simulink model "sm_car_testrig_susp_dwa_hp"  (R2025b)
settings: Solver=ode23t  StartTime=0.0  StopTime=1e-9  RelTol=1e-3  EnableMultiTasking=on
PostLoadFcn:
  | sm_car_load_vehicle_data(bdroot,'016');
undefined symbols (not defined in the file): Init, LAf, LAr, UAf, UAr, Vehicle, X, Y, Z
libraries: sm_lib x102, nesl_utility x67, Suspension_Utilities x8, Linkage_Arms x6, Linkage_DW_A x4, fl_lib x4, Linkage_Shock x2, Linkage_Uprights x2
(part 4 of 4)

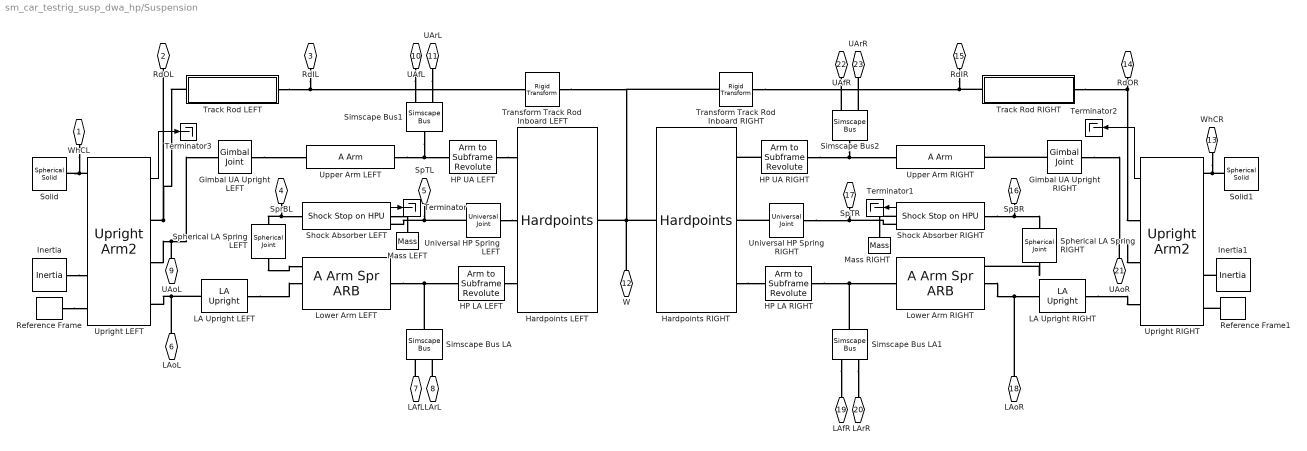
== system sm_car_testrig_susp_dwa_hp/Suspension ==
  Gimbal UA Upright LEFT : sm_lib/Joints/Gimbal Joint  JointMode=Normal  CompositeWrenchDir=FollowerOnBase  CompositeWrenchFrame=BaseFrame  SenseConstraintForce=off  SenseConstraintTorque=off  SenseTotalForce=off  SenseTotalTorque=off  RxPositionTargetSpecify=off  RxPositionTargetPriority=High  RxPositionTargetValue=0  RxPositionTargetValueUnits=deg  RxVelocityTargetSpecify=off  RxVelocityTargetPriority=High  RxVelocityTargetValue=0  RxVelocityTargetValueUnits=deg/s  RxEquilibriumPosition=0  RxEquilibriumPositionUnits=deg  RxSpringStiffness=0  RxSpringStiffnessUnits=N*m/deg  RxDampingCoefficient=0  RxDampingCoefficientUnits=N*m/(deg/s)  RxLowerLimitSpecify=off  RxLowerLimitBound=-90  RxLowerLimitBoundUnits=deg  RxLowerLimitStiffness=1e4  RxLowerLimitStiffnessUnits=N*m/deg  RxLowerLimitDamping=10  RxLowerLimitDampingUnits=N*m/(deg/s)  RxLowerLimitTransitionRegionWidth=0.1  RxLowerLimitTransitionRegionWidthUnits=deg  RxUpperLimitSpecify=off  RxUpperLimitBound=90  RxUpperLimitBoundUnits=deg  RxUpperLimitStiffness=1e4  RxUpperLimitStiffnessUnits=N*m/deg  RxUpperLimitDamping=10  RxUpperLimitDampingUnits=N*m/(deg/s)  RxUpperLimitTransitionRegionWidth=0.1  RxUpperLimitTransitionRegionWidthUnits=deg  RxTorqueActuationMode=NoTorque  RxMotionActuationMode=ComputedMotion  RxSensePosition=off  RxSenseVelocity=off  RxSenseAcceleration=off  RxSenseTorqueForce=off  RxSenseLowerLimitTorqueForce=off  RxSenseUpperLimitTorqueForce=off  RyPositionTargetSpecify=off  RyPositionTargetPriority=Low  RyPositionTargetValue=0  RyPositionTargetValueUnits=deg  RyVelocityTargetSpecify=off  RyVelocityTargetPriority=High  RyVelocityTargetValue=0  RyVelocityTargetValueUnits=deg/s  RyEquilibriumPosition=0  RyEquilibriumPositionUnits=deg  RySpringStiffness=0  RySpringStiffnessUnits=N*m/deg  RyDampingCoefficient=0  RyDampingCoefficientUnits=N*m/(deg/s)  RyLowerLimitSpecify=off  RyLowerLimitBound=-90  RyLowerLimitBoundUnits=deg  RyLowerLimitStiffness=1e4  RyLowerLimitStiffnessUnits=N*m/deg  RyLowerLimitDamping=10  RyLowerLimitDampingUnits=N*m/(deg/s)  RyLowerLimitTransitionRegionWidth=0.1  RyLowerLimitTransitionRegionWidthUnits=deg  RyUpperLimitSpecify=off  RyUpperLimitBound=90  RyUpperLimitBoundUnits=deg  RyUpperLimitStiffness=1e4  RyUpperLimitStiffnessUnits=N*m/deg  RyUpperLimitDamping=10  RyUpperLimitDampingUnits=N*m/(deg/s)  RyUpperLimitTransitionRegionWidth=0.1  RyUpperLimitTransitionRegionWidthUnits=deg  RyTorqueActuationMode=NoTorque  RyMotionActuationMode=ComputedMotion  RySensePosition=off  RySenseVelocity=off  RySenseAcceleration=off  RySenseTorqueForce=off  RySenseLowerLimitTorqueForce=off  RySenseUpperLimitTorqueForce=off  RzPositionTargetSpecify=off  RzPositionTargetPriority=Low  RzPositionTargetValue=90  RzPositionTargetValueUnits=deg  RzVelocityTargetSpecify=off  RzVelocityTargetPriority=High  RzVelocityTargetValue=0  RzVelocityTargetValueUnits=deg/s  RzEquilibriumPosition=0  RzEquilibriumPositionUnits=deg  RzSpringStiffness=0  RzSpringStiffnessUnits=N*m/deg  RzDampingCoefficient=0  RzDampingCoefficientUnits=N*m/(deg/s)  RzLowerLimitSpecify=off  RzLowerLimitBound=-90  RzLowerLimitBoundUnits=deg  RzLowerLimitStiffness=1e4  RzLowerLimitStiffnessUnits=N*m/deg  RzLowerLimitDamping=10  RzLowerLimitDampingUnits=N*m/(deg/s)  RzLowerLimitTransitionRegionWidth=0.1  RzLowerLimitTransitionRegionWidthUnits=deg  RzUpperLimitSpecify=off  RzUpperLimitBound=90  RzUpperLimitBoundUnits=deg  RzUpperLimitStiffness=1e4  RzUpperLimitStiffnessUnits=N*m/deg  RzUpperLimitDamping=10  RzUpperLimitDampingUnits=N*m/(deg/s)  RzUpperLimitTransitionRegionWidth=0.1  RzUpperLimitTransitionRegionWidthUnits=deg  RzTorqueActuationMode=NoTorque  RzMotionActuationMode=ComputedMotion  RzSensePosition=off  RzSenseVelocity=off  RzSenseAcceleration=off  RzSenseTorqueForce=off  RzSenseLowerLimitTorqueForce=off  RzSenseUpperLimitTorqueForce=off
  Gimbal UA Upright RIGHT : sm_lib/Joints/Gimbal Joint  JointMode=Normal  CompositeWrenchDir=FollowerOnBase  CompositeWrenchFrame=BaseFrame  SenseConstraintForce=off  SenseConstraintTorque=off  SenseTotalForce=off  SenseTotalTorque=off  RxPositionTargetSpecify=off  RxPositionTargetPriority=High  RxPositionTargetValue=0  RxPositionTargetValueUnits=deg  RxVelocityTargetSpecify=off  RxVelocityTargetPriority=High  RxVelocityTargetValue=0  RxVelocityTargetValueUnits=deg/s  RxEquilibriumPosition=0  RxEquilibriumPositionUnits=deg  RxSpringStiffness=0  RxSpringStiffnessUnits=N*m/deg  RxDampingCoefficient=0  RxDampingCoefficientUnits=N*m/(deg/s)  RxLowerLimitSpecify=off  RxLowerLimitBound=-90  RxLowerLimitBoundUnits=deg  RxLowerLimitStiffness=1e4  RxLowerLimitStiffnessUnits=N*m/deg  RxLowerLimitDamping=10  RxLowerLimitDampingUnits=N*m/(deg/s)  RxLowerLimitTransitionRegionWidth=0.1  RxLowerLimitTransitionRegionWidthUnits=deg  RxUpperLimitSpecify=off  RxUpperLimitBound=90  RxUpperLimitBoundUnits=deg  RxUpperLimitStiffness=1e4  RxUpperLimitStiffnessUnits=N*m/deg  RxUpperLimitDamping=10  RxUpperLimitDampingUnits=N*m/(deg/s)  RxUpperLimitTransitionRegionWidth=0.1  RxUpperLimitTransitionRegionWidthUnits=deg  RxTorqueActuationMode=NoTorque  RxMotionActuationMode=ComputedMotion  RxSensePosition=off  RxSenseVelocity=off  RxSenseAcceleration=off  RxSenseTorqueForce=off  RxSenseLowerLimitTorqueForce=off  RxSenseUpperLimitTorqueForce=off  RyPositionTargetSpecify=off  RyPositionTargetPriority=Low  RyPositionTargetValue=0  RyPositionTargetValueUnits=deg  RyVelocityTargetSpecify=off  RyVelocityTargetPriority=High  RyVelocityTargetValue=0  RyVelocityTargetValueUnits=deg/s  RyEquilibriumPosition=0  RyEquilibriumPositionUnits=deg  RySpringStiffness=0  RySpringStiffnessUnits=N*m/deg  RyDampingCoefficient=0  RyDampingCoefficientUnits=N*m/(deg/s)  RyLowerLimitSpecify=off  RyLowerLimitBound=-90  RyLowerLimitBoundUnits=deg  RyLowerLimitStiffness=1e4  RyLowerLimitStiffnessUnits=N*m/deg  RyLowerLimitDamping=10  RyLowerLimitDampingUnits=N*m/(deg/s)  RyLowerLimitTransitionRegionWidth=0.1  RyLowerLimitTransitionRegionWidthUnits=deg  RyUpperLimitSpecify=off  RyUpperLimitBound=90  RyUpperLimitBoundUnits=deg  RyUpperLimitStiffness=1e4  RyUpperLimitStiffnessUnits=N*m/deg  RyUpperLimitDamping=10  RyUpperLimitDampingUnits=N*m/(deg/s)  RyUpperLimitTransitionRegionWidth=0.1  RyUpperLimitTransitionRegionWidthUnits=deg  RyTorqueActuationMode=NoTorque  RyMotionActuationMode=ComputedMotion  RySensePosition=off  RySenseVelocity=off  RySenseAcceleration=off  RySenseTorqueForce=off  RySenseLowerLimitTorqueForce=off  RySenseUpperLimitTorqueForce=off  RzPositionTargetSpecify=off  RzPositionTargetPriority=Low  RzPositionTargetValue=90  RzPositionTargetValueUnits=deg  RzVelocityTargetSpecify=off  RzVelocityTargetPriority=High  RzVelocityTargetValue=0  RzVelocityTargetValueUnits=deg/s  RzEquilibriumPosition=0  RzEquilibriumPositionUnits=deg  RzSpringStiffness=0  RzSpringStiffnessUnits=N*m/deg  RzDampingCoefficient=0  RzDampingCoefficientUnits=N*m/(deg/s)  RzLowerLimitSpecify=off  RzLowerLimitBound=-90  RzLowerLimitBoundUnits=deg  RzLowerLimitStiffness=1e4  RzLowerLimitStiffnessUnits=N*m/deg  RzLowerLimitDamping=10  RzLowerLimitDampingUnits=N*m/(deg/s)  RzLowerLimitTransitionRegionWidth=0.1  RzLowerLimitTransitionRegionWidthUnits=deg  RzUpperLimitSpecify=off  RzUpperLimitBound=90  RzUpperLimitBoundUnits=deg  RzUpperLimitStiffness=1e4  RzUpperLimitStiffnessUnits=N*m/deg  RzUpperLimitDamping=10  RzUpperLimitDampingUnits=N*m/(deg/s)  RzUpperLimitTransitionRegionWidth=0.1  RzUpperLimitTransitionRegionWidthUnits=deg  RzTorqueActuationMode=NoTorque  RzMotionActuationMode=ComputedMotion  RzSensePosition=off  RzSenseVelocity=off  RzSenseAcceleration=off  RzSenseTorqueForce=off  RzSenseLowerLimitTorqueForce=off  RzSenseUpperLimitTorqueForce=off
  HP LA LEFT : Suspension_Utilities/Arm to Subframe Revolute  VariantControl=Variant1  LabelModeActiveChoice=Rigid_1Rev  popup_leftRight=Left  hp_f=hp_in_f_la  hp_r=hp_in_r_la  Connection=Lower_Arm_to_Subframe  VariantLabel=Lower_Arm_to_Subframe.class.Value
      settings: AttributesFormatString=%<ActiveVariant>
  HP LA RIGHT : Suspension_Utilities/Arm to Subframe Revolute  VariantControl=Variant1  LabelModeActiveChoice=Rigid_1Rev  popup_leftRight=Left  hp_f=hp_in_f_la  hp_r=hp_in_r_la  Connection=Lower_Arm_to_Subframe  VariantLabel=Lower_Arm_to_Subframe.class.Value
      settings: AttributesFormatString=%<ActiveVariant>
  HP UA LEFT : Suspension_Utilities/Arm to Subframe Revolute  VariantControl=Variant1  LabelModeActiveChoice=Rigid_1Rev  popup_leftRight=Left  hp_f=hp_in_f_ua  hp_r=hp_in_r_ua  Connection=Upper_Arm_to_Subframe  VariantLabel=Upper_Arm_to_Subframe.class.Value
      settings: AttributesFormatString=%<ActiveVariant>
  HP UA RIGHT : Suspension_Utilities/Arm to Subframe Revolute  VariantControl=Variant1  LabelModeActiveChoice=Rigid_1Rev  popup_leftRight=Left  hp_f=hp_in_f_ua  hp_r=hp_in_r_ua  Connection=Upper_Arm_to_Subframe  VariantLabel=Upper_Arm_to_Subframe.class.Value
      settings: AttributesFormatString=%<ActiveVariant>
  Hardpoints LEFT : Linkage_DW_A/DoubleWishboneA/Hardpoints  popup_leftRight=Left  hp_in_f_ua=Linkage.UpperWishbone.sInboardF.Value  hp_in_r_ua=Linkage.UpperWishbone.sInboardR.Value  hp_in_f_la=Linkage.LowerWishbone.sInboardF.Value  hp_in_r_la=Linkage.LowerWishbone.sInboardR.Value  hp_spr_top=Linkage.Shock.sTop.Value  clr_hp=Visual.hp.clr  opc_hp=Visual.hp.opc  size_hp=Visual.hp.rad
  Hardpoints RIGHT : Linkage_DW_A/DoubleWishboneA/Hardpoints  popup_leftRight=Right  hp_in_f_ua=Linkage.UpperWishbone.sInboardF.Value  hp_in_r_ua=Linkage.UpperWishbone.sInboardR.Value  hp_in_f_la=Linkage.LowerWishbone.sInboardF.Value  hp_in_r_la=Linkage.LowerWishbone.sInboardR.Value  hp_spr_top=Linkage.Shock.sTop.Value  clr_hp=Visual.hp.clr  opc_hp=Visual.hp.opc  size_hp=Visual.hp.rad
  Inertia : fl_lib/Mechanical/Rotational Elements/Inertia  inertia=0.01 kg*m^2  num_ports=foundation.enum.numPorts2.one  w_specify=on  w_priority=None  w=0 rad/s  w_nominal_specify=off  w_nominal_value=1  w_nominal_unit=rad/s  t_specify=off  t_priority=None  t=0 N*m  t_nominal_specify=off  t_nominal_value=1  t_nominal_unit=N*m
  Inertia1 : fl_lib/Mechanical/Rotational Elements/Inertia  inertia=0.01 kg*m^2  num_ports=foundation.enum.numPorts2.one  w_specify=on  w_priority=None  w=0 rad/s  w_nominal_specify=off  w_nominal_value=1  w_nominal_unit=rad/s  t_specify=off  t_priority=None  t=0 N*m  t_nominal_specify=off  t_nominal_value=1  t_nominal_unit=N*m
  LA Upright LEFT : Linkage_DW_A/DoubleWishboneA/LA Upright  SystemSampleTime=-1  VariantControl=Variant1  LabelModeActiveChoice=Steer  VariantActivationTime=update diagram  EmptyChoice=off  PassThrough=off  PassThroughVariantControl=(default)  EmptyChoiceVariantControl=(default)  AllowFlexibleInterface=on  Latency=0  AutoFrameSizeCalculation=off
      settings: AttributesFormatString=%<ActiveVariant>
  LA Upright RIGHT : Linkage_DW_A/DoubleWishboneA/LA Upright  SystemSampleTime=-1  VariantControl=Variant1  LabelModeActiveChoice=Steer  VariantActivationTime=update diagram  EmptyChoice=off  PassThrough=off  PassThroughVariantControl=(default)  EmptyChoiceVariantControl=(default)  AllowFlexibleInterface=on  Latency=0  AutoFrameSizeCalculation=off
      settings: AttributesFormatString=%<ActiveVariant>
  Lower Arm LEFT : Linkage_Arms/A Arm Spr ARB  popup_leftRight=Left  hp_in_f=Linkage.LowerWishbone.sInboardF.Value  hp_in_r=Linkage.LowerWishbone.sInboardR.Value  hp_out=Linkage.LowerWishbone.sOutboard.Value  hp_spr=Linkage.Shock.sBottom.Value  hp_arb=hp_arb  arm_mass=la_mass  clr_arm=clr_la  opc_arm=opc_la  radius_arm=radius_la
  Lower Arm RIGHT : Linkage_Arms/A Arm Spr ARB  popup_leftRight=Right  hp_in_f=Linkage.LowerWishbone.sInboardF.Value  hp_in_r=Linkage.LowerWishbone.sInboardR.Value  hp_out=Linkage.LowerWishbone.sOutboard.Value  hp_spr=Linkage.Shock.sBottom.Value  hp_arb=hp_arb  arm_mass=la_mass  clr_arm=clr_la  opc_arm=opc_la  radius_arm=radius_la
  Mass LEFT : fl_lib/Mechanical/Translational Elements/Mass  mass=1 kg  num_ports=foundation.enum.numPorts2.one  v_specify=off  v_priority=High  v=0 m/s  v_nominal_specify=off  v_nominal_value=1  v_nominal_unit=m/s  f_specify=off  f_priority=None  f=0 N  f_nominal_specify=off  f_nominal_value=1  f_nominal_unit=N
  Mass RIGHT : fl_lib/Mechanical/Translational Elements/Mass  mass=1 kg  num_ports=foundation.enum.numPorts2.one  v_specify=off  v_priority=High  v=0 m/s  v_nominal_specify=off  v_nominal_value=1  v_nominal_unit=m/s  f_specify=off  f_priority=None  f=0 N  f_nominal_specify=off  f_nominal_value=1  f_nominal_unit=N
  Reference Frame : sm_lib/Frames and Transforms/Reference Frame
  Reference Frame1 : sm_lib/Frames and Transforms/Reference Frame
  Shock Absorber LEFT : Linkage_Shock/Shock Stop on HPU  shock_pist_mass=Linkage.Shock.mPiston.Value  shock_cyl_mass=Linkage.Shock.mCylinder.Value  hp_spr_top=Linkage.Shock.sTop.Value  hp_spr_bot=Linkage.Shock.sBottom.Value  up_lim_bumpstop=Linkage.Endstop.xMax.Value  low_lim_bumpstop=Linkage.Endstop.xMin.Value  clr_conn_shock=Visual.hp.clr  opc_conn_shock=Visual.hp.opc  size_conn_shock=Visual.hp.rad  clr_shock_cyl=Visual.Shock.cyl.clr  opc_shock_cyl=Visual.part.opc  radius_shock_cyl=Visual.Shock.cyl.rad  clr_shock_piston=Visual.Shock.piston.clr  opc_shock_piston=Visual.part.opc  clr_shock_bumpstop=Visual.Shock.bumpstop.clr  opc_shock_bumpstop=Visual.part.opc  deadvol_len_shock_cyl=Visual.Shock.dead_length  piston_len_shock=Visual.Shock.piston.len  cyl_cap_len_shock=Visual.Shock.cap.len  bumpstop_len_shock=Visual.Shock.bumpstop.len
  Shock Absorber RIGHT : Linkage_Shock/Shock Stop on HPU  shock_pist_mass=Linkage.Shock.mPiston.Value  shock_cyl_mass=Linkage.Shock.mCylinder.Value  hp_spr_top=Linkage.Shock.sTop.Value  hp_spr_bot=Linkage.Shock.sBottom.Value  up_lim_bumpstop=Linkage.Endstop.xMax.Value  low_lim_bumpstop=Linkage.Endstop.xMin.Value  clr_conn_shock=Visual.hp.clr  opc_conn_shock=Visual.hp.opc  size_conn_shock=Visual.hp.rad  clr_shock_cyl=Visual.Shock.cyl.clr  opc_shock_cyl=Visual.part.opc  radius_shock_cyl=Visual.Shock.cyl.rad  clr_shock_piston=Visual.Shock.piston.clr  opc_shock_piston=Visual.part.opc  clr_shock_bumpstop=Visual.Shock.bumpstop.clr  opc_shock_bumpstop=Visual.part.opc  deadvol_len_shock_cyl=Visual.Shock.dead_length  piston_len_shock=Visual.Shock.piston.len  cyl_cap_len_shock=Visual.Shock.cap.len  bumpstop_len_shock=Visual.Shock.bumpstop.len
  Simscape Bus LA : SimscapeBus  HierarchyStrings=LAf;LAr
  Simscape Bus LA1 : SimscapeBus  HierarchyStrings=LAf;LAr
  Simscape Bus1 : SimscapeBus  HierarchyStrings=UAf;UAr
  Simscape Bus2 : SimscapeBus  HierarchyStrings=UAf;UAr
  Solid : sm_lib/Body Elements/Spherical Solid  SphereRadius=0.02  SphereRadiusUnits=m  ExportEntireGeometry=off  InertiaType=CalculateFromGeometry  BasedOnType=Density  Density=1000  DensityUnits=kg/m^3  Mass=1  MassUnits=kg  CenterOfMass=[0 0 0]  CenterOfMassUnits=m  MomentsOfInertia=[1 1 1]  MomentsOfInertiaUnits=kg*m^2  ProductsOfInertia=[0 0 0]  ProductsOfInertiaUnits=kg*m^2  GraphicType=FromGeometry  MarkerShape=Sphere  MarkerSize=10  GraphicVisPropType=SimpleVisualProperties  GraphicDiffuseColor=[0.5 0.5 0.5]  GraphicOpacity=1.0  GraphicSpecularColor=[0.5 0.5 0.5 1.0]  GraphicAmbientColor=[0.15 0.15 0.15 1.0]  GraphicEmissiveColor=[0.0 0.0 0.0 1.0]  GraphicShininess=75  DoExposeReferenceFrame=on  SerializedFrames=<Frames/>
  Solid1 : sm_lib/Body Elements/Spherical Solid  SphereRadius=0.02  SphereRadiusUnits=m  ExportEntireGeometry=off  InertiaType=CalculateFromGeometry  BasedOnType=Density  Density=1000  DensityUnits=kg/m^3  Mass=1  MassUnits=kg  CenterOfMass=[0 0 0]  CenterOfMassUnits=m  MomentsOfInertia=[1 1 1]  MomentsOfInertiaUnits=kg*m^2  ProductsOfInertia=[0 0 0]  ProductsOfInertiaUnits=kg*m^2  GraphicType=FromGeometry  MarkerShape=Sphere  MarkerSize=10  GraphicVisPropType=SimpleVisualProperties  GraphicDiffuseColor=[0.5 0.5 0.5]  GraphicOpacity=1.0  GraphicSpecularColor=[0.5 0.5 0.5 1.0]  GraphicAmbientColor=[0.15 0.15 0.15 1.0]  GraphicEmissiveColor=[0.0 0.0 0.0 1.0]  GraphicShininess=75  DoExposeReferenceFrame=on  SerializedFrames=<Frames/>
  Spherical LA Spring LEFT : sm_lib/Joints/Spherical Joint  JointMode=Normal  CompositeWrenchDir=FollowerOnBase  CompositeWrenchFrame=BaseFrame  SenseConstraintForce=off  SenseConstraintTorque=off  SenseTotalForce=off  SenseTotalTorque=off  PositionTargetSpecify=off  PositionTargetPriority=High  PositionTargetRotationMethod=None  PositionTargetFollAlignAxisA=+X  PositionTargetBaseAlignAxisA=+Y  PositionTargetFollAlignAxisB=+Y  PositionTargetBaseAlignAxisB=+Z  PositionTargetRotationStandardAxis=+Z  PositionTargetRotationAngle=0.0  PositionTargetRotationAngleUnits=deg  PositionTargetRotationArbitraryAxis=[0 0 1]  PositionTargetRotationSequenceAxes=FollowerAxes  PositionTargetRotationSequence=XYX  PositionTargetRotationSequenceAngles=[0 0 0]  PositionTargetRotationSequenceAnglesUnits=deg  PositionTargetRotationMatrix=[1 0 0; 0 1 0; 0 0 1]  PositionTargetQuaternion=[1 0 0 0]  VelocityTargetSpecify=off  VelocityTargetPriority=High  VelocityTargetValue=[0 0 0]  VelocityTargetValueUnits=deg/s  VelocityTargetInFollowerFrame=on  EqPosRotationMethod=None  EqPosFollAlignAxisA=+X  EqPosBaseAlignAxisA=+Y  EqPosFollAlignAxisB=+Y  EqPosBaseAlignAxisB=+Z  EqPosRotationStandardAxis=+Z  EqPosRotationAngle=0.0  EqPosRotationAngleUnits=deg  EqPosRotationArbitraryAxis=[0 0 1]  EqPosRotationSequenceAxes=FollowerAxes  EqPosRotationSequence=XYX  EqPosRotationSequenceAngles=[0 0 0]  EqPosRotationSequenceAnglesUnits=deg  EqPosRotationMatrix=[1 0 0; 0 1 0; 0 0 1]  EqPosQuaternion=[1 0 0 0]  SpringStiffness=0  SpringStiffnessUnits=N*m/deg  DampingCoefficient=0  DampingCoefficientUnits=N*m/(deg/s)  LowerLimitSpecify=off  LowerLimitBound=15  LowerLimitBoundUnits=deg  LowerLimitStiffness=1e4  LowerLimitStiffnessUnits=N*m/deg  LowerLimitDamping=10  LowerLimitDampingUnits=N*m/(deg/s)  LowerLimitTransitionRegionWidth=0.1  LowerLimitTransitionRegionWidthUnits=deg  UpperLimitSpecify=off  UpperLimitBound=45  UpperLimitBoundUnits=deg  UpperLimitStiffness=1e4  UpperLimitStiffnessUnits=N*m/deg  UpperLimitDamping=10  UpperLimitDampingUnits=N*m/(deg/s)  UpperLimitTransitionRegionWidth=0.1  UpperLimitTransitionRegionWidthUnits=deg  TorqueActuationMode=NoTorque  ActuateTorqueX=off  ActuateTorqueY=off  ActuateTorqueZ=off  ActuateTorque=off  ActuationFrame=BaseFrame  SensePosition=off  SenseVelocityX=off  SenseVelocityY=off  SenseVelocityZ=off  SenseVelocity=off  SenseAccelerationX=off  SenseAccelerationY=off  SenseAccelerationZ=off  SenseAcceleration=off  SenseLowerLimitTorqueMag=off  SenseUpperLimitTorqueMag=off  SensingFrame=BaseFrame
  Spherical LA Spring RIGHT : sm_lib/Joints/Spherical Joint  JointMode=Normal  CompositeWrenchDir=FollowerOnBase  CompositeWrenchFrame=BaseFrame  SenseConstraintForce=off  SenseConstraintTorque=off  SenseTotalForce=off  SenseTotalTorque=off  PositionTargetSpecify=off  PositionTargetPriority=High  PositionTargetRotationMethod=None  PositionTargetFollAlignAxisA=+X  PositionTargetBaseAlignAxisA=+Y  PositionTargetFollAlignAxisB=+Y  PositionTargetBaseAlignAxisB=+Z  PositionTargetRotationStandardAxis=+Z  PositionTargetRotationAngle=0.0  PositionTargetRotationAngleUnits=deg  PositionTargetRotationArbitraryAxis=[0 0 1]  PositionTargetRotationSequenceAxes=FollowerAxes  PositionTargetRotationSequence=XYX  PositionTargetRotationSequenceAngles=[0 0 0]  PositionTargetRotationSequenceAnglesUnits=deg  PositionTargetRotationMatrix=[1 0 0; 0 1 0; 0 0 1]  PositionTargetQuaternion=[1 0 0 0]  VelocityTargetSpecify=off  VelocityTargetPriority=High  VelocityTargetValue=[0 0 0]  VelocityTargetValueUnits=deg/s  VelocityTargetInFollowerFrame=on  EqPosRotationMethod=None  EqPosFollAlignAxisA=+X  EqPosBaseAlignAxisA=+Y  EqPosFollAlignAxisB=+Y  EqPosBaseAlignAxisB=+Z  EqPosRotationStandardAxis=+Z  EqPosRotationAngle=0.0  EqPosRotationAngleUnits=deg  EqPosRotationArbitraryAxis=[0 0 1]  EqPosRotationSequenceAxes=FollowerAxes  EqPosRotationSequence=XYX  EqPosRotationSequenceAngles=[0 0 0]  EqPosRotationSequenceAnglesUnits=deg  EqPosRotationMatrix=[1 0 0; 0 1 0; 0 0 1]  EqPosQuaternion=[1 0 0 0]  SpringStiffness=0  SpringStiffnessUnits=N*m/deg  DampingCoefficient=0  DampingCoefficientUnits=N*m/(deg/s)  LowerLimitSpecify=off  LowerLimitBound=15  LowerLimitBoundUnits=deg  LowerLimitStiffness=1e4  LowerLimitStiffnessUnits=N*m/deg  LowerLimitDamping=10  LowerLimitDampingUnits=N*m/(deg/s)  LowerLimitTransitionRegionWidth=0.1  LowerLimitTransitionRegionWidthUnits=deg  UpperLimitSpecify=off  UpperLimitBound=45  UpperLimitBoundUnits=deg  UpperLimitStiffness=1e4  UpperLimitStiffnessUnits=N*m/deg  UpperLimitDamping=10  UpperLimitDampingUnits=N*m/(deg/s)  UpperLimitTransitionRegionWidth=0.1  UpperLimitTransitionRegionWidthUnits=deg  TorqueActuationMode=NoTorque  ActuateTorqueX=off  ActuateTorqueY=off  ActuateTorqueZ=off  ActuateTorque=off  ActuationFrame=BaseFrame  SensePosition=off  SenseVelocityX=off  SenseVelocityY=off  SenseVelocityZ=off  SenseVelocity=off  SenseAccelerationX=off  SenseAccelerationY=off  SenseAccelerationZ=off  SenseAcceleration=off  SenseLowerLimitTorqueMag=off  SenseUpperLimitTorqueMag=off  SensingFrame=BaseFrame
  Terminator{,1..3} (4 alike) : Terminator
  Track Rod LEFT : Subsystem  Variant=on  VariantControlMode=label  VariantControl=Steer  LabelModeActiveChoice=Steer
      settings: AttributesFormatString=%<ActiveVariant>
      mask Display: disp(' ');
  Track Rod RIGHT : Subsystem  Variant=on  VariantControlMode=label  VariantControl=Steer  LabelModeActiveChoice=Steer
      settings: AttributesFormatString=%<ActiveVariant>
      mask Display: disp(' ');
  Transform Track Rod Inboard LEFT : sm_lib/Frames and Transforms/Rigid Transform  RotationMethod=None  FollAlignAxisA=+X  BaseAlignAxisA=+Y  FollAlignAxisB=+Y  BaseAlignAxisB=+Z  RotationStandardAxis=+Z  RotationAngle=0.0  RotationAngleUnits=deg  RotationArbitraryAxis=[0 0 1]  RotationSequenceAxes=FollowerAxes  RotationSequence=XYX  RotationSequenceAngles=[0 0 0]  RotationSequenceAnglesUnits=deg  RotationMatrix=[1 0 0; 0 1 0; 0 0 1]  Quaternion=[1 0 0 0]  TranslationMethod=Cartesian  TranslationCartesianOffset=Linkage.TrackRod.sInboard.Value  TranslationCartesianOffsetUnits=m  TranslationStandardAxis=+Z  TranslationStandardOffset=0  TranslationStandardOffsetUnits=m  TranslationROffset=0  TranslationROffsetUnits=m  TranslationThetaOffset=0  TranslationThetaOffsetUnits=deg  TranslationZOffset=0  TranslationZOffsetUnits=m
  Transform Track Rod Inboard RIGHT : sm_lib/Frames and Transforms/Rigid Transform  RotationMethod=None  FollAlignAxisA=+X  BaseAlignAxisA=+Y  FollAlignAxisB=+Y  BaseAlignAxisB=+Z  RotationStandardAxis=+Z  RotationAngle=0.0  RotationAngleUnits=deg  RotationArbitraryAxis=[0 0 1]  RotationSequenceAxes=FollowerAxes  RotationSequence=XYX  RotationSequenceAngles=[0 0 0]  RotationSequenceAnglesUnits=deg  RotationMatrix=[1 0 0; 0 1 0; 0 0 1]  Quaternion=[1 0 0 0]  TranslationMethod=Cartesian  TranslationCartesianOffset=Linkage.TrackRod.sInboard.Value.*[1 -1 1]  TranslationCartesianOffsetUnits=m  TranslationStandardAxis=+Z  TranslationStandardOffset=0  TranslationStandardOffsetUnits=m  TranslationROffset=0  TranslationROffsetUnits=m  TranslationThetaOffset=0  TranslationThetaOffsetUnits=deg  TranslationZOffset=0  TranslationZOffsetUnits=m
  Universal HP Spring LEFT : sm_lib/Joints/Universal Joint  JointMode=Normal  CompositeWrenchDir=FollowerOnBase  CompositeWrenchFrame=BaseFrame  SenseConstraintForce=off  SenseConstraintTorque=off  SenseTotalForce=off  SenseTotalTorque=off  RxPositionTargetSpecify=off  RxPositionTargetPriority=High  RxPositionTargetValue=0  RxPositionTargetValueUnits=deg  RxVelocityTargetSpecify=off  RxVelocityTargetPriority=High  RxVelocityTargetValue=0  RxVelocityTargetValueUnits=deg/s  RxEquilibriumPosition=0  RxEquilibriumPositionUnits=deg  RxSpringStiffness=0  RxSpringStiffnessUnits=N*m/deg  RxDampingCoefficient=0  RxDampingCoefficientUnits=N*m/(deg/s)  RxLowerLimitSpecify=off  RxLowerLimitBound=-90  RxLowerLimitBoundUnits=deg  RxLowerLimitStiffness=1e4  RxLowerLimitStiffnessUnits=N*m/deg  RxLowerLimitDamping=10  RxLowerLimitDampingUnits=N*m/(deg/s)  RxLowerLimitTransitionRegionWidth=0.1  RxLowerLimitTransitionRegionWidthUnits=deg  RxUpperLimitSpecify=off  RxUpperLimitBound=90  RxUpperLimitBoundUnits=deg  RxUpperLimitStiffness=1e4  RxUpperLimitStiffnessUnits=N*m/deg  RxUpperLimitDamping=10  RxUpperLimitDampingUnits=N*m/(deg/s)  RxUpperLimitTransitionRegionWidth=0.1  RxUpperLimitTransitionRegionWidthUnits=deg  RxTorqueActuationMode=NoTorque  RxMotionActuationMode=ComputedMotion  RxSensePosition=off  RxSenseVelocity=off  RxSenseAcceleration=off  RxSenseTorqueForce=off  RxSenseLowerLimitTorqueForce=off  RxSenseUpperLimitTorqueForce=off  RyPositionTargetSpecify=off  RyPositionTargetPriority=High  RyPositionTargetValue=0  RyPositionTargetValueUnits=deg  RyVelocityTargetSpecify=off  RyVelocityTargetPriority=High  RyVelocityTargetValue=0  RyVelocityTargetValueUnits=deg/s  RyEquilibriumPosition=0  RyEquilibriumPositionUnits=deg  RySpringStiffness=0  RySpringStiffnessUnits=N*m/deg  RyDampingCoefficient=0  RyDampingCoefficientUnits=N*m/(deg/s)  RyLowerLimitSpecify=off  RyLowerLimitBound=-90  RyLowerLimitBoundUnits=deg  RyLowerLimitStiffness=1e4  RyLowerLimitStiffnessUnits=N*m/deg  RyLowerLimitDamping=10  RyLowerLimitDampingUnits=N*m/(deg/s)  RyLowerLimitTransitionRegionWidth=0.1  RyLowerLimitTransitionRegionWidthUnits=deg  RyUpperLimitSpecify=off  RyUpperLimitBound=90  RyUpperLimitBoundUnits=deg  RyUpperLimitStiffness=1e4  RyUpperLimitStiffnessUnits=N*m/deg  RyUpperLimitDamping=10  RyUpperLimitDampingUnits=N*m/(deg/s)  RyUpperLimitTransitionRegionWidth=0.1  RyUpperLimitTransitionRegionWidthUnits=deg  RyTorqueActuationMode=NoTorque  RyMotionActuationMode=ComputedMotion  RySensePosition=off  RySenseVelocity=off  RySenseAcceleration=off  RySenseTorqueForce=off  RySenseLowerLimitTorqueForce=off  RySenseUpperLimitTorqueForce=off
  Universal HP Spring RIGHT : sm_lib/Joints/Universal Joint  JointMode=Normal  CompositeWrenchDir=FollowerOnBase  CompositeWrenchFrame=BaseFrame  SenseConstraintForce=off  SenseConstraintTorque=off  SenseTotalForce=off  SenseTotalTorque=off  RxPositionTargetSpecify=off  RxPositionTargetPriority=High  RxPositionTargetValue=0  RxPositionTargetValueUnits=deg  RxVelocityTargetSpecify=off  RxVelocityTargetPriority=High  RxVelocityTargetValue=0  RxVelocityTargetValueUnits=deg/s  RxEquilibriumPosition=0  RxEquilibriumPositionUnits=deg  RxSpringStiffness=0  RxSpringStiffnessUnits=N*m/deg  RxDampingCoefficient=0  RxDampingCoefficientUnits=N*m/(deg/s)  RxLowerLimitSpecify=off  RxLowerLimitBound=-90  RxLowerLimitBoundUnits=deg  RxLowerLimitStiffness=1e4  RxLowerLimitStiffnessUnits=N*m/deg  RxLowerLimitDamping=10  RxLowerLimitDampingUnits=N*m/(deg/s)  RxLowerLimitTransitionRegionWidth=0.1  RxLowerLimitTransitionRegionWidthUnits=deg  RxUpperLimitSpecify=off  RxUpperLimitBound=90  RxUpperLimitBoundUnits=deg  RxUpperLimitStiffness=1e4  RxUpperLimitStiffnessUnits=N*m/deg  RxUpperLimitDamping=10  RxUpperLimitDampingUnits=N*m/(deg/s)  RxUpperLimitTransitionRegionWidth=0.1  RxUpperLimitTransitionRegionWidthUnits=deg  RxTorqueActuationMode=NoTorque  RxMotionActuationMode=ComputedMotion  RxSensePosition=off  RxSenseVelocity=off  RxSenseAcceleration=off  RxSenseTorqueForce=off  RxSenseLowerLimitTorqueForce=off  RxSenseUpperLimitTorqueForce=off  RyPositionTargetSpecify=off  RyPositionTargetPriority=High  RyPositionTargetValue=0  RyPositionTargetValueUnits=deg  RyVelocityTargetSpecify=off  RyVelocityTargetPriority=High  RyVelocityTargetValue=0  RyVelocityTargetValueUnits=deg/s  RyEquilibriumPosition=0  RyEquilibriumPositionUnits=deg  RySpringStiffness=0  RySpringStiffnessUnits=N*m/deg  RyDampingCoefficient=0  RyDampingCoefficientUnits=N*m/(deg/s)  RyLowerLimitSpecify=off  RyLowerLimitBound=-90  RyLowerLimitBoundUnits=deg  RyLowerLimitStiffness=1e4  RyLowerLimitStiffnessUnits=N*m/deg  RyLowerLimitDamping=10  RyLowerLimitDampingUnits=N*m/(deg/s)  RyLowerLimitTransitionRegionWidth=0.1  RyLowerLimitTransitionRegionWidthUnits=deg  RyUpperLimitSpecify=off  RyUpperLimitBound=90  RyUpperLimitBoundUnits=deg  RyUpperLimitStiffness=1e4  RyUpperLimitStiffnessUnits=N*m/deg  RyUpperLimitDamping=10  RyUpperLimitDampingUnits=N*m/(deg/s)  RyUpperLimitTransitionRegionWidth=0.1  RyUpperLimitTransitionRegionWidthUnits=deg  RyTorqueActuationMode=NoTorque  RyMotionActuationMode=ComputedMotion  RySensePosition=off  RySenseVelocity=off  RySenseAcceleration=off  RySenseTorqueForce=off  RySenseLowerLimitTorqueForce=off  RySenseUpperLimitTorqueForce=off
  Upper Arm LEFT : Linkage_Arms/A Arm  popup_leftRight=Left  hp_in_f=Linkage.UpperWishbone.sInboardF.Value  hp_in_r=Linkage.UpperWishbone.sInboardR.Value  hp_out=Linkage.UpperWishbone.sOutboard.Value  arm_mass=ua_mass  clr_arm=clr_ua  opc_arm=opc_ua  radius_arm=radius_ua
  Upper Arm RIGHT : Linkage_Arms/A Arm  popup_leftRight=Right  hp_in_f=Linkage.UpperWishbone.sInboardF.Value  hp_in_r=Linkage.UpperWishbone.sInboardR.Value  hp_out=Linkage.UpperWishbone.sOutboard.Value  arm_mass=ua_mass  clr_arm=clr_ua  opc_arm=opc_ua  radius_arm=radius_ua
  Upright LEFT : Linkage_Uprights/Upright Arm2  popup_leftRight=Left  hp_ua_out=Linkage.UpperWishbone.sOutboard.Value  hp_la_out=Linkage.LowerWishbone.sOutboard.Value  hp_upr_rod=Linkage.TrackRod.sOutboard.Value  hp_upr_cg=Linkage.Upright.sCG.Value  hp_upr_wc=Linkage.Upright.sWheelCentre.Value  axle_len=Linkage.Upright.xAxle.Value  axle_whlc_to_bearing=Linkage.Upright.xWCtoBearing.Value  axle_mass=Linkage.Upright.mAxle.Value  atoe=Linkage.Upright.aToe.Value  acamber=Linkage.Upright.aCamber.Value  upr_mass=Linkage.Upright.m.Value  whl_init_spd_upr=Init.Axle1.nWheel.Value(1)  clr_conn_upr=Visual.hp.clr  opc_conn_upr=Visual.hp.opc  size_conn_upr=Visual.hp.rad  clr_upr=Visual.Upright.clr  opc_upr=Visual.part.opc  radius_upr=Visual.Upright.rad  clr_axle=Visual.Axle.clr  opc_axle=Visual.part.opc  radius_axle=Visual.Axle.rad
  Upright RIGHT : Linkage_Uprights/Upright Arm2  popup_leftRight=Right  hp_ua_out=Linkage.UpperWishbone.sOutboard.Value  hp_la_out=Linkage.LowerWishbone.sOutboard.Value  hp_upr_rod=Linkage.TrackRod.sOutboard.Value  hp_upr_cg=Linkage.Upright.sCG.Value  hp_upr_wc=Linkage.Upright.sWheelCentre.Value  axle_len=Linkage.Upright.xAxle.Value  axle_whlc_to_bearing=Linkage.Upright.xWCtoBearing.Value  axle_mass=Linkage.Upright.mAxle.Value  atoe=Linkage.Upright.aToe.Value  acamber=Linkage.Upright.aCamber.Value  upr_mass=Linkage.Upright.m.Value  whl_init_spd_upr=Init.Axle1.nWheel.Value(2)  clr_conn_upr=Visual.hp.clr  opc_conn_upr=Visual.hp.opc  size_conn_upr=Visual.hp.rad  clr_upr=Visual.Upright.clr  opc_upr=Visual.part.opc  radius_upr=Visual.Upright.rad  clr_axle=Visual.Axle.clr  opc_axle=Visual.part.opc  radius_axle=Visual.Axle.rad
  WhCL : PMIOPort  Side=Left
  RdOL : PMIOPort  Port=2  Side=Left
  RdIL : PMIOPort  Port=3  Side=Left
  SprBL : PMIOPort  Port=4  Side=Left
  SpTL : PMIOPort  Port=5  Side=Left
  LAoL : PMIOPort  Port=6  Side=Left
  LAfL : PMIOPort  Port=7  Side=Left
  LArL : PMIOPort  Port=8  Side=Left
  UAoL : PMIOPort  Port=9  Side=Left
  UAfL : PMIOPort  Port=10  Side=Left
  UArL : PMIOPort  Port=11  Side=Left
  W : PMIOPort  Port=12  Side=Left
  WhCR : PMIOPort  Port=13  Side=Right
  RdOR : PMIOPort  Port=14  Side=Right
  RdIR : PMIOPort  Port=15  Side=Right
  SpBR : PMIOPort  Port=16  Side=Right
  SpTR : PMIOPort  Port=17  Side=Right
  LAoR : PMIOPort  Port=18  Side=Right
  LAfR : PMIOPort  Port=19  Side=Right
  LArR : PMIOPort  Port=20  Side=Right
  UAoR : PMIOPort  Port=21  Side=Right
  UAfR : PMIOPort  Port=22  Side=Right
  UArR : PMIOPort  Port=23  Side=Right
  wires:
  Shock Absorber LEFT/1 -> Terminator/1
  Shock Absorber RIGHT/1 -> Terminator1/1
  Upright RIGHT/1 -> Terminator2/1
  Upright LEFT/1 -> Terminator3/1
  connections:
  HP LA LEFT/LConn1 -- Hardpoints LEFT/LConn3
  LA Upright LEFT/LConn1 -- Lower Arm LEFT/LConn2
  SprBL/RConn1 -- Spherical LA Spring LEFT/RConn1 -- Shock Absorber LEFT/LConn1
  Universal HP Spring RIGHT/LConn1 -- Hardpoints RIGHT/LConn2
  Simscape Bus LA1/LConn1 -- LAfR/RConn1
  Transform Track Rod Inboard RIGHT/RConn1 -- Track Rod RIGHT/RConn1 -- RdIR/RConn1
  HP LA RIGHT/RConn1 -- Lower Arm RIGHT/RConn1 -- Simscape Bus LA1/RConn1
  Upright LEFT/RConn2 -- Gimbal UA Upright LEFT/LConn1 -- UAoL/RConn1
  Transform Track Rod Inboard RIGHT/LConn1 -- Transform Track Rod Inboard LEFT/LConn1 -- Hardpoints LEFT/RConn1 -- W/RConn1 -- Hardpoints RIGHT/RConn1
  LA Upright RIGHT/RConn1 -- Upright RIGHT/RConn3
  Spherical LA Spring LEFT/LConn1 -- Lower Arm LEFT/LConn1
  RdOR/RConn1 -- Track Rod RIGHT/LConn1 -- Upright RIGHT/RConn1
  Universal HP Spring LEFT/LConn1 -- Hardpoints LEFT/LConn2
  Solid1/RConn1 -- WhCR/RConn1 -- Upright RIGHT/LConn1
  Lower Arm LEFT/RConn1 -- HP LA LEFT/RConn1 -- Simscape Bus LA/RConn1
  Universal HP Spring LEFT/RConn1 -- SpTL/RConn1 -- Shock Absorber LEFT/RConn2
  Lower Arm RIGHT/LConn2 -- LAoR/RConn1 -- LA Upright RIGHT/LConn1
  Simscape Bus2/LConn1 -- UAfR/RConn1
  UAfL/RConn1 -- Simscape Bus1/LConn1
  Gimbal UA Upright LEFT/RConn1 -- Upper Arm LEFT/LConn1
  Simscape Bus2/LConn2 -- UArR/RConn1
  Upright LEFT/LConn1 -- WhCL/RConn1 -- Solid/RConn1
  Gimbal UA Upright RIGHT/RConn1 -- Upper Arm RIGHT/LConn1
  Universal HP Spring RIGHT/RConn1 -- Shock Absorber RIGHT/RConn2 -- SpTR/RConn1
  HP UA LEFT/LConn1 -- Hardpoints LEFT/LConn1
  Spherical LA Spring RIGHT/LConn1 -- Lower Arm RIGHT/LConn1
  HP UA RIGHT/LConn1 -- Hardpoints RIGHT/LConn1
  HP UA RIGHT/RConn1 -- Simscape Bus2/RConn1 -- Upper Arm RIGHT/RConn1
  Upper Arm LEFT/RConn1 -- Simscape Bus1/RConn1 -- HP UA LEFT/RConn1
  LA Upright LEFT/RConn1 -- LAoL/RConn1 -- Upright LEFT/RConn3
  SpBR/RConn1 -- Shock Absorber RIGHT/LConn1 -- Spherical LA Spring RIGHT/RConn1
  Gimbal UA Upright RIGHT/LConn1 -- UAoR/RConn1 -- Upright RIGHT/RConn2
  Hardpoints RIGHT/LConn3 -- HP LA RIGHT/LConn1
  Simscape Bus LA1/LConn2 -- LArR/RConn1
  LArL/RConn1 -- Simscape Bus LA/LConn2
  LAfL/RConn1 -- Simscape Bus LA/LConn1
  UArL/RConn1 -- Simscape Bus1/LConn2
  Shock Absorber LEFT/RConn1 -- Mass LEFT/LConn1
  Shock Absorber RIGHT/RConn1 -- Mass RIGHT/LConn1
  Upright LEFT/RConn1 -- Track Rod LEFT/LConn1 -- RdOL/RConn1
  RdIL/RConn1 -- Transform Track Rod Inboard LEFT/RConn1 -- Track Rod LEFT/RConn1
  Inertia/LConn1 -- Upright LEFT/LConn4
  Reference Frame/RConn1 -- Upright LEFT/LConn5
  Inertia1/LConn1 -- Upright RIGHT/LConn4
  Reference Frame1/RConn1 -- Upright RIGHT/LConn5

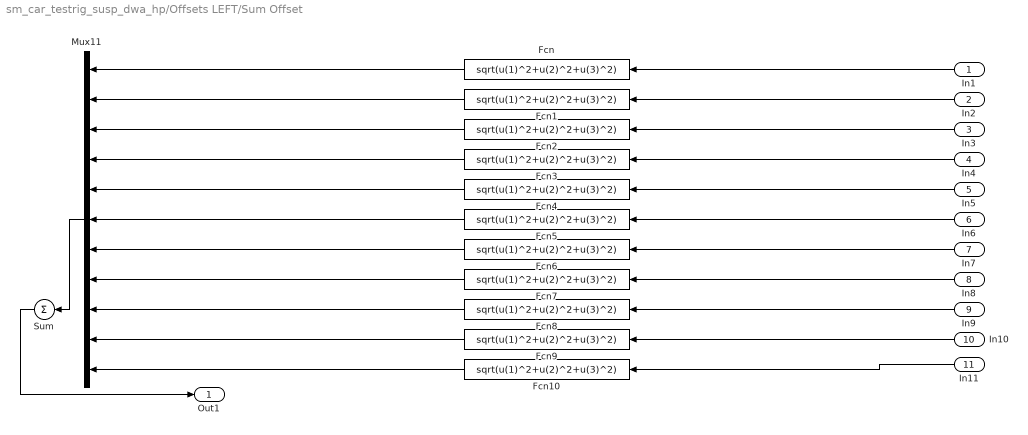
== system sm_car_testrig_susp_dwa_hp/Offsets LEFT/Sum Offset ==
  In1 : Inport
  In2 : Inport  Port=2
  In3 : Inport  Port=3
  In4 : Inport  Port=4
  In5 : Inport  Port=5
  In6 : Inport  Port=6
  In7 : Inport  Port=7
  In8 : Inport  Port=8
  In9 : Inport  Port=9
  In10 : Inport  Port=10
  In11 : Inport  Port=11
  Fcn{,1..10} (11 alike) : Fcn  Expr=sqrt(u(1)^2+u(2)^2+u(3)^2)
  Mux11 : Mux  Inputs=11
  Sum : Sum  Inputs=+
  Out1 : Outport  VectorParamsAs1DForOutWhenUnconnected=off
  wires:
  Mux11/1 -> Sum/1
  Sum/1 -> Out1/1
  In1/1 -> Fcn/1
  In2/1 -> Fcn1/1
  In3/1 -> Fcn2/1
  In4/1 -> Fcn3/1
  In5/1 -> Fcn4/1
  In6/1 -> Fcn5/1
  In7/1 -> Fcn6/1
  In8/1 -> Fcn7/1
  In9/1 -> Fcn8/1
  In10/1 -> Fcn9/1
  In11/1 -> Fcn10/1
  Fcn/1 -> Mux11/1
  Fcn1/1 -> Mux11/2
  Fcn2/1 -> Mux11/3
  Fcn3/1 -> Mux11/4
  Fcn4/1 -> Mux11/5
  Fcn5/1 -> Mux11/6
  Fcn6/1 -> Mux11/7
  Fcn7/1 -> Mux11/8
  Fcn8/1 -> Mux11/9
  Fcn9/1 -> Mux11/10
  Fcn10/1 -> Mux11/11

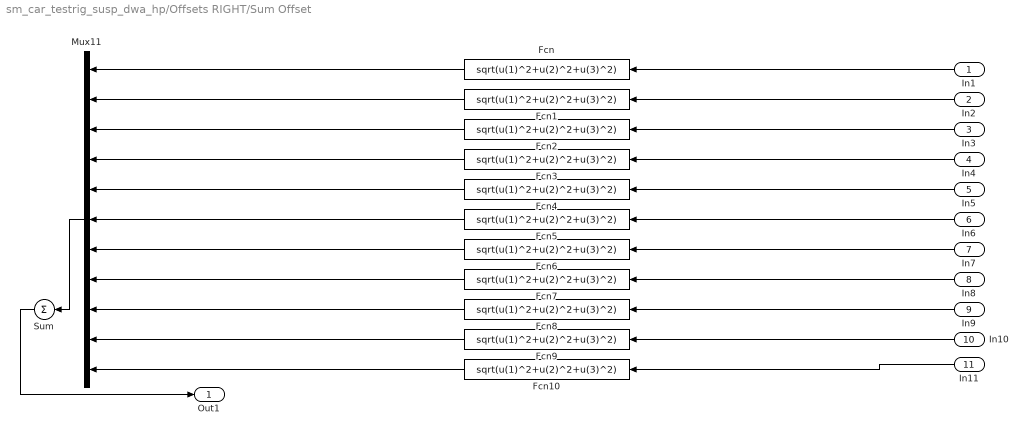
== system sm_car_testrig_susp_dwa_hp/Offsets RIGHT/Sum Offset ==
  In1 : Inport
  In2 : Inport  Port=2
  In3 : Inport  Port=3
  In4 : Inport  Port=4
  In5 : Inport  Port=5
  In6 : Inport  Port=6
  In7 : Inport  Port=7
  In8 : Inport  Port=8
  In9 : Inport  Port=9
  In10 : Inport  Port=10
  In11 : Inport  Port=11
  Fcn{,1..10} (11 alike) : Fcn  Expr=sqrt(u(1)^2+u(2)^2+u(3)^2)
  Mux11 : Mux  Inputs=11
  Sum : Sum  Inputs=+
  Out1 : Outport  VectorParamsAs1DForOutWhenUnconnected=off
  wires:
  Fcn10/1 -> Mux11/11
  Fcn9/1 -> Mux11/10
  Fcn8/1 -> Mux11/9
  Fcn7/1 -> Mux11/8
  Fcn6/1 -> Mux11/7
  Fcn5/1 -> Mux11/6
  Fcn4/1 -> Mux11/5
  Fcn3/1 -> Mux11/4
  Fcn2/1 -> Mux11/3
  Fcn1/1 -> Mux11/2
  Fcn/1 -> Mux11/1
  In11/1 -> Fcn10/1
  In10/1 -> Fcn9/1
  In9/1 -> Fcn8/1
  In8/1 -> Fcn7/1
  In7/1 -> Fcn6/1
  In6/1 -> Fcn5/1
  In5/1 -> Fcn4/1
  In4/1 -> Fcn3/1
  In3/1 -> Fcn2/1
  In2/1 -> Fcn1/1
  In1/1 -> Fcn/1
  Sum/1 -> Out1/1
  Mux11/1 -> Sum/1

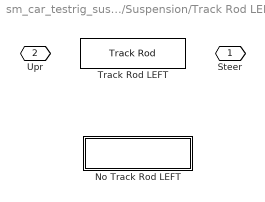
== system sm_car_testrig_susp_dwa_hp/Suspension/Track Rod LEFT ==
  No Track Rod LEFT : Subsystem  VariantControl=No_Steer
  Track Rod LEFT : Linkage_Arms/Track Rod  VariantControl=Steer  popup_leftRight=Left  hp_in=Linkage.TrackRod.sInboard.Value  hp_out=Linkage.TrackRod.sOutboard.Value  rod_mass=Linkage.TrackRod.m.Value  clr_conn_rod=Visual.hp.clr  opc_conn_rod=Visual.hp.opc  size_conn_rod=Visual.hp.rad  clr_rod=Visual.TrackRod.clr  opc_rod=Visual.part.opc  radius_rod=Visual.TrackRod.rad
  "  Steer" : PMIOPort  Side=Right
  " Upr" : PMIOPort  Port=2  Side=Left

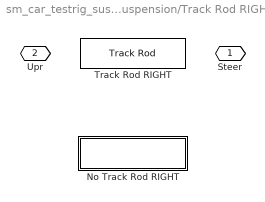
== system sm_car_testrig_susp_dwa_hp/Suspension/Track Rod RIGHT ==
  No Track Rod RIGHT : Subsystem  VariantControl=No_Steer
  Track Rod RIGHT : Linkage_Arms/Track Rod  VariantControl=Steer  popup_leftRight=Right  hp_in=Linkage.TrackRod.sInboard.Value  hp_out=Linkage.TrackRod.sOutboard.Value  rod_mass=Linkage.TrackRod.m.Value  clr_conn_rod=Visual.hp.clr  opc_conn_rod=Visual.hp.opc  size_conn_rod=Visual.hp.rad  clr_rod=Visual.TrackRod.clr  opc_rod=Visual.part.opc  radius_rod=Visual.TrackRod.rad
  "  Steer" : PMIOPort  Side=Right
  " Upr" : PMIOPort  Port=2  Side=Left

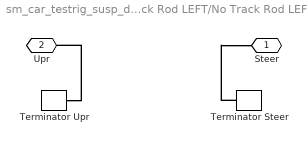
== system sm_car_testrig_susp_dwa_hp/Suspension/Track Rod LEFT/No Track Rod LEFT ==
  Terminator Steer : Suspension_Utilities/Terminator  SystemSampleTime=-1  VariantActivationTime=update diagram  EmptyChoice=off  PassThrough=off  PassThroughVariantControl=(default)  EmptyChoiceVariantControl=(default)  AllowFlexibleInterface=on  Latency=0  AutoFrameSizeCalculation=off
  Terminator Upr : Suspension_Utilities/Terminator  SystemSampleTime=-1  VariantActivationTime=update diagram  EmptyChoice=off  PassThrough=off  PassThroughVariantControl=(default)  EmptyChoiceVariantControl=(default)  AllowFlexibleInterface=on  Latency=0  AutoFrameSizeCalculation=off
  " Steer" : PMIOPort  Side=Right
  Upr : PMIOPort  Port=2  Side=Left
  connections:
  Terminator Upr/RConn1 -- Upr/RConn1
  Terminator Steer/RConn1 -- " Steer"/RConn1

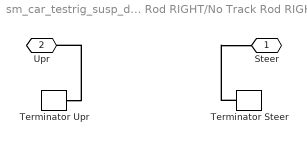
== system sm_car_testrig_susp_dwa_hp/Suspension/Track Rod RIGHT/No Track Rod RIGHT ==
  Terminator Steer : Suspension_Utilities/Terminator  SystemSampleTime=-1  VariantActivationTime=update diagram  EmptyChoice=off  PassThrough=off  PassThroughVariantControl=(default)  EmptyChoiceVariantControl=(default)  AllowFlexibleInterface=on  Latency=0  AutoFrameSizeCalculation=off
  Terminator Upr : Suspension_Utilities/Terminator  SystemSampleTime=-1  VariantActivationTime=update diagram  EmptyChoice=off  PassThrough=off  PassThroughVariantControl=(default)  EmptyChoiceVariantControl=(default)  AllowFlexibleInterface=on  Latency=0  AutoFrameSizeCalculation=off
  " Steer" : PMIOPort  Side=Right
  Upr : PMIOPort  Port=2  Side=Left
  connections:
  Terminator Steer/RConn1 -- " Steer"/RConn1
  Terminator Upr/RConn1 -- Upr/RConn1
